simulink model "W1_P8"  (R2020b)
settings: Solver=VariableStepAuto  StartTime=0.0  StopTime=10.0  RelTol=1e-3
settings Model: Creator=ADMIN  LastModifiedBy=ADMIN

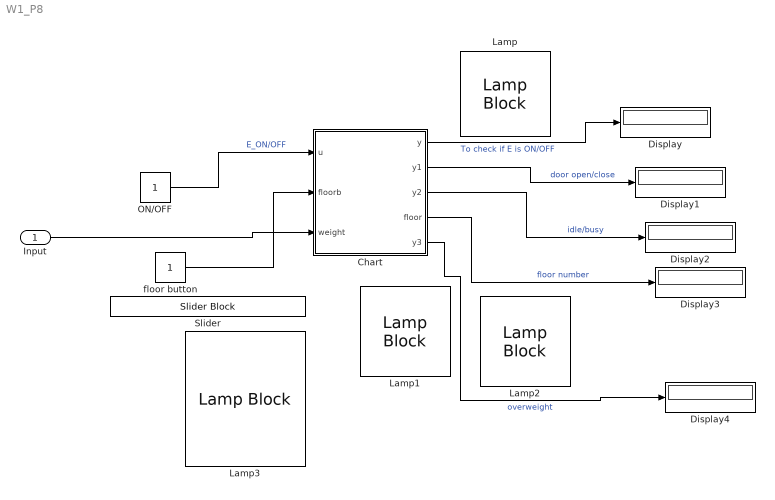
== system W1_P8 ==
  Input : Inport
  Chart : Stateflow chart  TreatAsAtomicUnit=on
  Display{,1..4} (5 alike) : Display
  Lamp{,1..3} (4 alike) : LampBlock
  ON/OFF : Constant
  Slider : SliderBlock  ScaleMax=5  TickInterval=1
  floor button : Constant
  wires:
  Chart/2(y1) -> Display1/1  "door open/close"
  Chart/1(y) -> Display/1  "To check if E is ON/OFF"
  Input/1 -> Chart/3(weight)
  Chart/3(y2) -> Display2/1  "idle/busy"
  ON/OFF/1 -> Chart/1(u)  "E_ON/OFF"
  floor button/1 -> Chart/2(floorb)
  Chart/4(floor) -> Display3/1  "floor number"
  Chart/5(y3) -> Display4/1  "overweight"

== stateflow chart W1_P8/Chart ==
  state Elevator_on
    entry: y=1;
    y3=0;
    note: [floorb<floor]{y1= 1 }
    state DOWN
      entry:
      floor=floor-1;
    state Delay1
      entry:
      floor=floor-1;
    state Idle_state
      entry: y1=0;
    state UP
      entry:
      floor=floor+1;
    state Delay
      entry:
      floor=floor+1;
    state Door_open1
      entry:
      y2=1;
    state Door_close1
      entry:
      y2=0;
    state Door_open
      entry:
      y2=1;
    state Door_close
      entry:
      y2=0;
    (default) -> Idle_state
    DOWN -> Delay1 [order 1] : [floorb<floor]
    Idle_state -> DOWN [order 2]
    Delay1 -> DOWN [order 1] : [floorb<floor]
    Idle_state -> UP [order 1] : [floorb>floor]{y1=1}
    DOWN -> Door_open1 [order 2] : [floorb==floor]
    Delay1 -> Door_open1 [order 2] : [floor==floorb]
    Delay -> UP [order 1] : [floorb>floor]
    UP -> Delay [order 1] : [floorb>floor]
    Door_open1 -> Door_close1 : [after(5,sec)]
    UP -> Door_open [order 2] : [floorb==floor]
    Delay -> Door_open [order 2] : [floor==floorb]
    Door_open -> Door_close : [after(5,sec)]
  state overload
    entry: y3=1;
  state Elevator_off
    entry: y=0;
  (default) -> Elevator_on
  Elevator_on -> overload [order 2] : [weight>500]
  overload -> Elevator_on : [weight<500]
  Elevator_on -> Elevator_off [order 1] : [u==0]
  Elevator_off -> Elevator_on : [u==1]
  data: u input; y output [0..1]; floorb input; y1 output [0..1]; y2 output [0..1]; floor output [0..5] =0; weight input; y3 output
